simulink model "TOP_LEVEL_SIM"  (R2019b)
settings: Solver=FixedStepAuto  StartTime=0.0  StopTime=2  FixedStep=Tsim  MaxStep=Tsim  RelTol=1e-3
PreLoadFcn:
  | Ts = 1/20000;
  | Tsim = Ts/10;
libraries: simulink x2, powerlib_meascontrol x1
settings Model: Creator=Nathan Petersen  LastModifiedBy=npetersen2
settings OptimizationCC: DefaultParameterBehavior=Inlined  GainParamInheritBuiltInType=on  UseFloatMulNetSlope=on  UseSpecifiedMinMax=on  InlineInvariantSignals=on  StrengthReduction=on  PassReuseOutputArgsAs=Individual arguments  ZeroExternalMemoryAtStartup=off  ZeroInternalMemoryAtStartup=off  NoFixptDivByZeroProtection=on  EfficientFloat2IntCast=on  LifeSpan=1  OptimizeBlockOrder=speed  OptimizationPriority=Speed  OptimizationCustomize=off  MultiThreadedLoops=on  EfficientTunableParamExpr=on
settings DebuggingCC: ParameterTunabilityLossMsg=error  UniqueDataStoreMsg=warning
settings HardwareCC: ProdLongLongMode=on
settings ModelReferenceCC: ModelReferenceNumInstancesAllowed=Single
settings SFSimCC: MATLABDynamicMemAlloc=off
settings RTWCC: SystemTargetFile=ert.tlc  GenCodeOnly=on  TemplateMakefile=ert_default_tmf  GenerateReport=on  BuildConfiguration=Faster Runs  LaunchReport=on  GenerateCodeMetricsReport=on
settings CodeAppCC: ForceParamTrailComments=on  IgnoreCustomStorageClasses=off  IgnoreTestpoints=on  MaxIdLength=50  OperatorAnnotations=on  SimulinkDataObjDesc=on  SFDataObjDesc=on  InsertBlockDesc=on
settings ERTTargetCC: TargetLangStandard=C99 (ISO)  CombineSignalStateStructs=on  SuppressErrorStatus=on  SupportNonFinite=off  InlinedParameterPlacement=NonHierarchical  ERTCustomFileTemplate=example_file_process.tlc

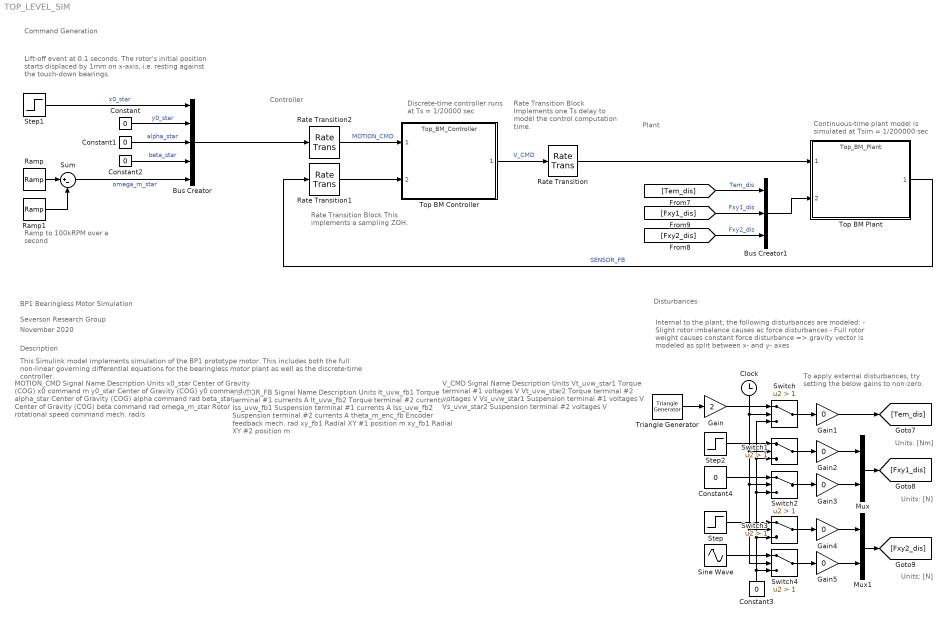
== system TOP_LEVEL_SIM ==
  note: Continuous-time plant model is simulated at Tsim = 1/200000 sec
  note: Units: [N]
  note: SENSOR_FB
      |
      | Signal Name
      | Description
      | Units
      |
      | It_uvw_fb1
      | Torque terminal #1 currents
      | A
      |
      | It_uvw_fb2
      | Torque terminal #2 currents
      | A
      |
      | Iss_uvw_fb1
      | Suspension terminal #1 currents
      | A
      |
      | Iss_uvw_fb2
      | Suspension terminal #2 currents
      | A
      |
      | theta_m_enc_fb
      | Encoder feedback
      | mech. rad
      |
      | xy_fb1
      | Radial XY #1 position
      | m
      |
      | xy_fb1
      | Radial XY #2 position
      | m
  note: Internal to the plant, the following disturbances are modeled:
      | - Slight rotor imbalance causes ac force disturbances
      | - Full rotor weight causes constant force disturbance
      |     => gravity vector is modeled as split between x- and y- axes
  note: To apply external disturbances, try setting the below gains to non-zero.
  note: Lift-off event at 0.1 seconds.
      | The rotor's initial position starts displaced by 1mm on x-axis, i.e. resting against the touch-down bearings.
  note: Ramp to 100kRPM over a second
  note: Description
  note: November 2020
  note: Severson Research Group
  note: BP1 Bearingless Motor Simulation
  note: This Simulink model implements simulation of the BP1 prototype motor. This includes both the full non-linear governing differential equations for the bearingless motor plant as well as the discrete-time controller.
  note: Plant
  note: Disturbances
  note: Rate Transition Block
      | This implements a sampling ZOH.
  note: Rate Transition Block
      | Implements one Ts delay to model the control computation time.
  note: Command Generation
  note: Controller
  note: Units: [N]
  note: Units: [Nm]
  note: V_CMD
      |
      | Signal Name
      | Description
      | Units
      |
      | Vt_uvw_star1
      | Torque terminal #1 voltages
      | V
      |
      | Vt_uvw_star2
      | Torque terminal #2 voltages
      | V
      |
      | Vs_uvw_star1
      | Suspension terminal #1 voltages
      | V
      |
      | Vs_uvw_star2
      | Suspension terminal #2 voltages
      | V
  note: MOTION_CMD
      |
      | Signal Name
      | Description
      | Units
      |
      | x0_star
      | Center of Gravity (COG) x0 command
      | m
      |
      | y0_star
      | Center of Gravity (COG) y0 command
      | m
      |
      | alpha_star
      | Center of Gravity (COG) alpha command
      | rad
      |
      | beta_star
      | Center of Gravity (COG) beta command
      | rad
      |
      | omega_m_star
      | Rotor rotational speed command
      | mech. rad/s
  note: Discrete-time controller runs at Ts = 1/20000 sec
  Bus Creator : BusCreator  Inputs=5
  Bus Creator1 : BusCreator  Inputs=3
  Clock : Clock
  Constant{,1..4} (5 alike) : Constant  Value=0
  Gain : Gain  Gain=2
  Gain{1..5} (5 alike) : Gain  Gain=0
  Mux : Mux  Inputs=2
  Mux1 : Mux  Inputs=2
  Ramp : simulink/Sources/Ramp  slope=((100e3/60)*2*pi) / 1  start=0.5  InitialOutput=0
  Ramp1 : simulink/Sources/Ramp  slope=((100e3/60)*2*pi) / 1  start=1.5  InitialOutput=0
  Rate Transition : RateTransition  OutPortSampleTime=Tsim
  Rate Transition1 : RateTransition  OutPortSampleTime=Ts
  Rate Transition2 : RateTransition  OutPortSampleTime=Ts
  Sine Wave : Sin  Amplitude=10  Frequency=2*pi*10  SampleTime=0
  Step : Step  After=10  SampleTime=0
  Step1 : Step  Time=0.1  Before=-1*1e-3  After=0  SampleTime=0
  Step2 : Step  After=-10  SampleTime=0
  Sum : Sum  Inputs=|+-
  Switch{,1..4} (5 alike) : Switch  Criteria=u2 > Threshold  Threshold=1
  Top BM Controller : ModelReference  ModelNameDialog=Top_BM_Controller  ModelReferenceVersion=1.2025
  Top BM Plant : ModelReference  ModelNameDialog=Top_BM_Plant  ModelReferenceVersion=1.2029
  Triangle Generator : powerlib_meascontrol/Pulse & Signal Generators/Triangle Generator  Freq=10  Phase=90  Ts=0
  wires:
  Top BM Plant/1 -> Rate Transition1/1  "SENSOR_FB"
  Bus Creator1/1 -> Top BM Plant/2
  [Tem_dis] -> Bus Creator1/1  "Tem_dis"
  [Fxy1_dis] -> Bus Creator1/2  "Fxy1_dis"
  [Fxy2_dis] -> Bus Creator1/3  "Fxy2_dis"
  Switch/1 -> Gain1/1
  Mux/1 -> [Fxy1_dis]
  Switch1/1 -> Gain2/1
  Mux1/1 -> [Fxy2_dis]
  Top BM Controller/1 -> Rate Transition/1  "V_CMD"
  Rate Transition/1 -> Top BM Plant/1
  Rate Transition1/1 -> Top BM Controller/2
  Constant/1 -> Bus Creator/2  "y0_star"
  Constant2/1 -> Bus Creator/4  "beta_star"
  Sum/1 -> Bus Creator/5  "omega_m_star"
  Step1/1 -> Bus Creator/1  "x0_star"
  Constant1/1 -> Bus Creator/3  "alpha_star"
  Bus Creator/1 -> Rate Transition2/1
  Ramp/1 -> Sum/1
  Ramp1/1 -> Sum/2
  Switch2/1 -> Gain3/1
  Switch4/1 -> Gain5/1
  Switch3/1 -> Gain4/1
  Clock/1 -> Switch4/2, Switch3/2, Switch2/2, Switch1/2, Switch/2
  Constant3/1 -> Switch2/3, Switch/3, Switch1/3, Switch3/3, Switch4/3
  Step/1 -> Switch3/1
  Sine Wave/1 -> Switch4/1
  Triangle Generator/1 -> Gain/1
  Gain/1 -> Switch/1
  Step2/1 -> Switch1/1
  Constant4/1 -> Switch2/1
  Gain1/1 -> [Tem_dis]
  Gain2/1 -> Mux/1
  Gain3/1 -> Mux/2
  Gain4/1 -> Mux1/1
  Gain5/1 -> Mux1/2
  Rate Transition2/1 -> Top BM Controller/1  "MOTION_CMD"
